simulink library "mpc555drivers"  (Simulink 6.0)
settings: Solver=ode45  SolverMode=SingleTasking  StartTime=0.0  StopTime=10.0  RelTol=1e-3
PreLoadFcn:
  | RTWConfigurationCB('preloadfcn', bdroot);
InitFcn:
  | % START RTW CONFIGURATION CODE %
  | RTWConfigurationCB('rtw_target_initfcn',gcs);
  | % END RTW CONFIGURATION CODE %
undefined symbols (not defined in the file or in its folder): pmax, scale
libraries: passthrough x52, driver_interface_library x18, mpc555toucan x11, mpc555extras x9, config_library x7, exprofilelib x4, simulink x3, mpc555drivers x2, canblocks x1
(part 3 of 3)

== system mpc555drivers/Time Processor Unit (TPU3)/TPU3 Digital In/Process Simulation Input ==
  SimIn : Inport  Port=1  LatchInput=off
  Constant : Constant  Value=0
  Data Type Conversion1 : DataTypeConversion  SaturateOnIntegerOverflow=on  RndMeth=Zero
  Relational Operator : RelationalOperator  Operator=>  LogicOutDataTypeMode=Boolean  InputSameDT=on
  SimOut : Outport
  wires:
  SimIn/1 -> Relational Operator/1
  Data Type Conversion1/1 -> Relational Operator/2
  Relational Operator/1 -> SimOut/1
  Constant/1 -> Data Type Conversion1/1

== system mpc555drivers/Execution Profiling/MPC555 Execution Profiling via SCI1/Send Execution Profiling Data via Serial/Send data over serial ==
  In1 : Inport  Port=1  LatchInput=off
  Enable : EnablePort
  Constant : Constant  Value=8  OutDataTypeMode=uint32
  Serial Transmit : mpc555drivers/Serial Communications Interface (SCI)/Serial Transmit  module=1  show_length=on  show_num_sent=off  T=-1
  wires:
  Constant/1 -> Serial Transmit/2
  In1/1 -> Serial Transmit/1

== system mpc555drivers/Execution Profiling/MPC555 Execution Profiling via SCI1/Start Profiling/Start execution profiling ==
  Enable : EnablePort
  Execution Profiling Start : exprofilelib/Execution Profiling Start

== system mpc555drivers/Modular Input/Output System (MIOS1)/MIOS Digital Out/Subsystem/fd ==
  u : Inport  Port=1  LatchInput=off
  Bitwise Operator : simulink/Logic and Bit Operations/Bitwise Operator  logicop=OR  UseBitMask=off  BitMask=bin2dec('11011001')  BitMaskRealWorld=Stored Integer
  Bitwise Operator1 : simulink/Logic and Bit Operations/Bitwise Operator  logicop=AND  UseBitMask=on  BitMask=bitcmp(sum(masks,[],'double'),16)  BitMaskRealWorld=Stored Integer
  Constant : Constant  Value=0  OutDataTypeMode=uint16
  Mux : Mux  Inputs=2
  RTW memory get : driver_interface_library/Input Driver  t=t  expr='MIOS1.MPIOSM32DR.R '  portWidth=1  pOpt=[]  expression_type=Expression
  RTW memory set : driver_interface_library/Output Driver  operation_type=Generic Code  input_is_contiguous=off  t=-1  expr='MIOS1.MPIOSM32DR.R = (VUINT16) %<u>;'  port_width=-1  pOpt=[]
  Signal Specification : SignalSpecification  DataType=uint16
  Switch : Switch  Criteria=u2 > Threshold  SaturateOnIntegerOverflow=on  InputSameDT=on
  masks : Constant  Value=masks
  wires:
  Signal Specification/1 -> Bitwise Operator1/1
  masks/1 -> Switch/1
  RTW memory get/1 -> Signal Specification/1
  u/1 -> Switch/2
  Bitwise Operator/1 -> RTW memory set/1
  Constant/1 -> Switch/3
  Switch/1 -> Mux/1
  Mux/1 -> Bitwise Operator/1
  Bitwise Operator1/1 -> Mux/2

== system mpc555drivers/Queued Analog-To-Digital Converter Module-64/QADC Analog In/Process Simulation Input/Switch Case Action Subsystem2 ==
  In1 : Inport  Port=1  LatchInput=off
  Bitwise Operator : mpc555extras/Bitwise Operator  logicop=SHIFT LEFT  zeroTest=No Test  UseBitMask=on  BitMask=6  maskInBinary=off
  Constant : Constant  Value=uint16(2^9)
  Sum : Sum  Inputs=+-  InputSameDT=on
  Out1 : Outport
  wires:
  Bitwise Operator/1 -> Out1/1
  In1/1 -> Sum/1
  Sum/1 -> Bitwise Operator/1
  Constant/1 -> Sum/2
